simulink model "test_advanced_fuzzy"  (Simulink 4.00)
settings: Solver=FixedStepDiscrete  StartTime=0.0  StopTime=60  FixedStep=0.05  RelTol=1e-3
settings Model: LastModifiedBy=bsaunder

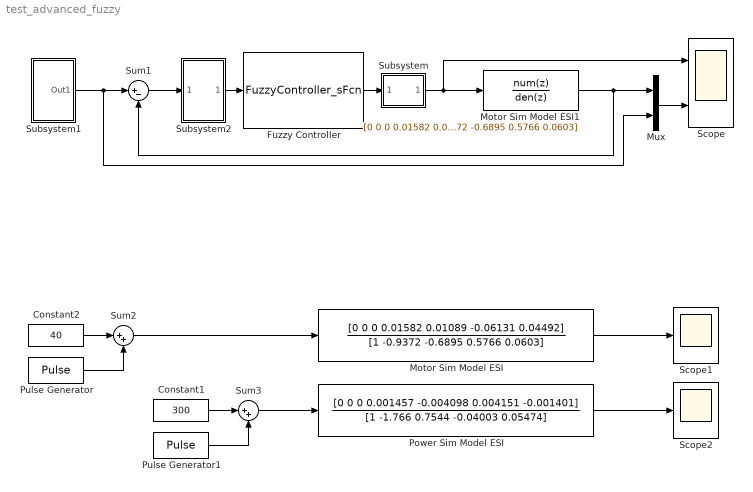
== system test_advanced_fuzzy ==
  Constant1 : Constant  Value=300
  Constant2 : Constant  Value=40
  Fuzzy Controller : S-Function  FunctionName=FuzzyController_sFcn  Parameters=[-0.5 -0.7 -1.0; -0.2 -0.4 -0.6; 0.1 0.0 -0.1; 0.6 0.4 0.2; 1.0 0.7 0.5]  PortCounts=[]  SFunctionModules=''
      mask Type: DAQ_AO
      mask Display:
      | plot([0.1 0.2 0.5 0.8; 0.2 0.5 0.8 0.9], [0.9 0.9 0.7 0.9; 0.9 0.7 0.9 0.9])
      | plot([0.1 0.2 0.5 0.8; 0.2 0.5 0.8 0.9], [0.7 0.7 0.9 0.7; 0.7 0.9 0.7 0.7])
      | 
      | text(0.5, 0.5, 'Fuzzy logic Controller', 'VerticalAlignment', 'middle','HorizontalAlignment','center');
      | 
      | plot([0.1 0.3 0.5 0.7; 0.3 0.5 0.7 0.9], [0.1 0.3 0.1 0.3; 0.3 0.1 0.3 0.1])
      | plot([0.3 0.5; 0.5 0.7 ], [0.1 0.3; 0.3 0.1])
  Motor Sim Model ESI : DiscreteFilter  Numerator=[0 0 0 0.01582 0.01089 -0.06131 0.04492]  Denominator=[1 -0.9372 -0.6895 0.5766 0.0603]  SampleTime=0.05  Realization=auto
      settings: RTWStateStorageClass=Auto
  Motor Sim Model ESI1 : DiscreteFilter  Numerator=[0 0 0 0.01582 0.01089 -0.06131 0.04492]  Denominator=[1 -0.9372 -0.6895 0.5766 0.0603]  SampleTime=0.05  Realization=auto
      settings: RTWStateStorageClass=Auto
  Mux : Mux  Inputs=2
  Power Sim Model ESI : DiscreteFilter  Numerator=[0 0 0 0.001457 -0.004098 0.004151 -0.001401]  Denominator=[1 -1.766 0.7544 -0.04003 0.05474]  SampleTime=0.05  Realization=auto
      settings: RTWStateStorageClass=Auto
  Pulse Generator : DiscretePulseGenerator  PulseType=Time-based  Amplitude=20  Period=40  PulseWidth=50  PhaseDelay=0  SampleTime=1
  Pulse Generator1 : DiscretePulseGenerator  PulseType=Time-based  Amplitude=200  Period=40  PulseWidth=50  PhaseDelay=0  SampleTime=1
  Scope : Scope  NumInputPorts=2
      settings: TimeRange=60  YMin=0~0  YMax=70~75  SaveToWorkspace=off  SaveName=ScopeData  LimitDataPoints=on  MaxDataPoints=5000
  Scope1 : Scope
      settings: TimeRange=60  YMin=0  YMax=70  SaveToWorkspace=off  SaveName=ScopeData3  LimitDataPoints=on  MaxDataPoints=5000
  Scope2 : Scope
      settings: TimeRange=60  YMin=0  YMax=70  SaveToWorkspace=off  SaveName=ScopeData4  LimitDataPoints=on  MaxDataPoints=5000
  Subsystem : Subsystem
      settings: RTWFcnNameOpts=Auto  RTWFileNameOpts=Auto
  Subsystem1 : Subsystem
      settings: RTWFcnNameOpts=Auto  RTWFileNameOpts=Auto
  Subsystem2 : Subsystem
      settings: RTWFcnNameOpts=Auto  RTWFileNameOpts=Auto
  Sum1 : Sum  Inputs=|+-  SaturateOnIntegerOverflow=on
  Sum2 : Sum  Inputs=|++  SaturateOnIntegerOverflow=on
  Sum3 : Sum  Inputs=|++  SaturateOnIntegerOverflow=on
  wires:
  Subsystem1/1(Out1) -> Mux/2, Sum1/1
  Fuzzy Controller/1 -> Subsystem/1(In1)
  Motor Sim Model ESI1/1 -> Mux/1, Sum1/2
  Mux/1 -> Scope/2
  Subsystem2/1(Out1) -> Fuzzy Controller/1
  Sum1/1 -> Subsystem2/1(In1)
  Subsystem/1(Out1) -> Scope/1, Motor Sim Model ESI1/1
  Constant2/1 -> Sum2/1
  Pulse Generator/1 -> Sum2/2
  Sum2/1 -> Motor Sim Model ESI/1
  Motor Sim Model ESI/1 -> Scope1/1
  Constant1/1 -> Sum3/1
  Pulse Generator1/1 -> Sum3/2
  Power Sim Model ESI/1 -> Scope2/1
  Sum3/1 -> Power Sim Model ESI/1

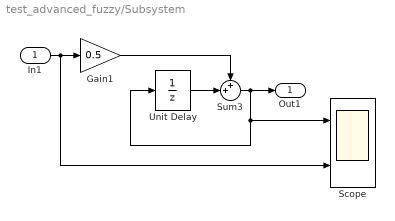
== system test_advanced_fuzzy/Subsystem ==
  In1 : Inport  Port=1  LatchInput=off
  Gain1 : Gain  Gain=0.5  Multiplication=Element-wise(K.*u)  SaturateOnIntegerOverflow=on
  Scope : Scope  NumInputPorts=2
      settings: TimeRange=60  YMin=0~-0.4  YMax=70~1  SaveToWorkspace=off  LimitDataPoints=on  MaxDataPoints=5000
  Sum3 : Sum  Inputs=++|  SaturateOnIntegerOverflow=on
  Unit Delay : UnitDelay  X0=0  SampleTime=0.05
      settings: RTWStateStorageClass=Auto
  Out1 : Outport  Port=1
  wires:
  In1/1 -> Gain1/1, Scope/2
  Sum3/1 -> Out1/1, Scope/1, Unit Delay/1
  Unit Delay/1 -> Sum3/2
  Gain1/1 -> Sum3/1

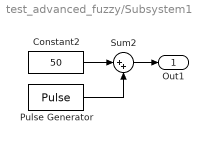
== system test_advanced_fuzzy/Subsystem1 ==
  Constant2 : Constant  Value=50
  Pulse Generator : DiscretePulseGenerator  PulseType=Time-based  Amplitude=20  Period=40  PulseWidth=50  PhaseDelay=0  SampleTime=1
  Sum2 : Sum  Inputs=|++  SaturateOnIntegerOverflow=on
  Out1 : Outport  Port=1
  wires:
  Constant2/1 -> Sum2/1
  Pulse Generator/1 -> Sum2/2
  Sum2/1 -> Out1/1

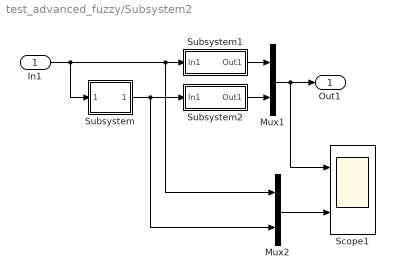
== system test_advanced_fuzzy/Subsystem2 ==
  In1 : Inport  Port=1  LatchInput=off
  Mux1 : Mux  Inputs=2
  Mux2 : Mux  Inputs=2
  Scope1 : Scope  NumInputPorts=2
      settings: TimeRange=60  YMin=-1~-600  YMax=1~1400  SaveToWorkspace=off  SaveName=ScopeData2  LimitDataPoints=on  MaxDataPoints=5000
  Subsystem : Subsystem
      settings: RTWFcnNameOpts=Auto  RTWFileNameOpts=Auto
  Subsystem1 : Subsystem
      settings: RTWFcnNameOpts=Auto  RTWFileNameOpts=Auto
  Subsystem2 : Subsystem
      settings: RTWFcnNameOpts=Auto  RTWFileNameOpts=Auto
  Out1 : Outport  Port=1
  wires:
  In1/1 -> Subsystem/1(In1), Subsystem1/1(In1), Mux2/1
  Subsystem/1(Out1) -> Subsystem2/1(In1), Mux2/2
  Mux1/1 -> Out1/1, Scope1/1
  Subsystem2/1(Out1) -> Mux1/2
  Subsystem1/1(Out1) -> Mux1/1
  Mux2/1 -> Scope1/2

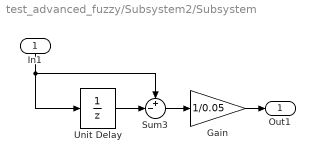
== system test_advanced_fuzzy/Subsystem2/Subsystem ==
  In1 : Inport  Orientation=down  Port=1  LatchInput=off
  Gain : Gain  Gain=1/0.05  Multiplication=Element-wise(K.*u)  SaturateOnIntegerOverflow=on
  Sum3 : Sum  Inputs=+-|  SaturateOnIntegerOverflow=on
  Unit Delay : UnitDelay  X0=0  SampleTime=0.05
      settings: RTWStateStorageClass=Auto
  Out1 : Outport  Port=1
  wires:
  Unit Delay/1 -> Sum3/2
  Sum3/1 -> Gain/1
  In1/1 -> Unit Delay/1, Sum3/1
  Gain/1 -> Out1/1

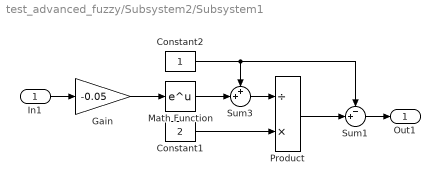
== system test_advanced_fuzzy/Subsystem2/Subsystem1 ==
  In1 : Inport  Port=1  LatchInput=off
  Constant1 : Constant  Value=2
  Constant2 : Constant  Value=1
  Gain : Gain  Gain=-0.05  Multiplication=Element-wise(K.*u)  SaturateOnIntegerOverflow=on
  Math Function : Math  Operator=exp  OutputSignalType=auto
  Product : Product  Inputs=/*  Multiplication=Element-wise(.*)  SaturateOnIntegerOverflow=on
  Sum1 : Sum  Inputs=-+|  SaturateOnIntegerOverflow=on
  Sum3 : Sum  Inputs=++|  SaturateOnIntegerOverflow=on
  Out1 : Outport  Port=1
  wires:
  Gain/1 -> Math Function/1
  Math Function/1 -> Sum3/2
  Constant2/1 -> Sum3/1, Sum1/1
  Constant1/1 -> Product/2
  Sum3/1 -> Product/1
  Product/1 -> Sum1/2
  In1/1 -> Gain/1
  Sum1/1 -> Out1/1

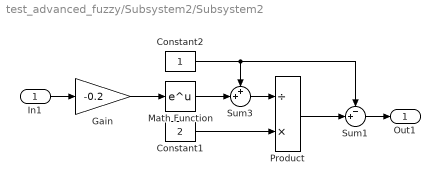
== system test_advanced_fuzzy/Subsystem2/Subsystem2 ==
  In1 : Inport  Port=1  LatchInput=off
  Constant1 : Constant  Value=2
  Constant2 : Constant  Value=1
  Gain : Gain  Gain=-0.2  Multiplication=Element-wise(K.*u)  SaturateOnIntegerOverflow=on
  Math Function : Math  Operator=exp  OutputSignalType=auto
  Product : Product  Inputs=/*  Multiplication=Element-wise(.*)  SaturateOnIntegerOverflow=on
  Sum1 : Sum  Inputs=-+|  SaturateOnIntegerOverflow=on
  Sum3 : Sum  Inputs=++|  SaturateOnIntegerOverflow=on
  Out1 : Outport  Port=1
  wires:
  Sum1/1 -> Out1/1
  In1/1 -> Gain/1
  Product/1 -> Sum1/2
  Sum3/1 -> Product/1
  Constant1/1 -> Product/2
  Constant2/1 -> Sum1/1, Sum3/1
  Math Function/1 -> Sum3/2
  Gain/1 -> Math Function/1
